simulink model "data_acquisition"  (R2023b)
settings: Solver=FixedStepDiscrete  StartTime=0.0  StopTime=Inf  RelTol=1e-3  EnableMultiTasking=on
libraries: c2802xlib x3
settings Model: SimulationMode=external  ExtModeTrigDuration=8  Creator=Yamukelani  LastModifiedBy=yamzi
settings SolverCC: AutoInsertRateTranBlk=on
settings DataIOCC: LoggingToFile=on  LoggingFileName=C:\Users\yamzi\source_code\msc_research\rul_prediction\src\datasets\msc_rul_data.mat
settings OptimizationCC: UseDivisionForNetSlopeComputation=on  GainParamInheritBuiltInType=on  UseFloatMulNetSlope=on  DefaultUnderspecifiedDataType=single  EnhancedBackFolding=on  PassReuseOutputArgsAs=Individual arguments  EfficientFloat2IntCast=on  MaxStackSize=768  OptimizeBlockOrder=speed  DifferentSizesBufferReuse=on  OptimizationCustomize=off  EfficientTunableParamExpr=on
settings DebuggingCC: ParameterTunabilityLossMsg=error
settings HardwareCC: ProdBitPerChar=16  ProdBitPerInt=16  ProdBitPerPointer=32  ProdBitPerSizeT=32  ProdBitPerPtrDiffT=32  ProdLargestAtomicInteger=Integer  ProdLargestAtomicFloat=None  ProdWordSize=16  ProdLongLongMode=on  ProdHWDeviceType=Texas Instruments->C2000  TargetBitPerPointer=64  TargetBitPerSizeT=64  TargetBitPerPtrDiffT=64  TargetLongLongMode=on  TargetIntDivRoundTo=Zero  TargetEndianess=LittleEndian  TargetWordSize=64  TargetHWDeviceType=MATLAB Host  ProdEqTarget=off
settings ModelReferenceCC: ModelReferenceNumInstancesAllowed=Single
settings SFSimCC: SimUserIncludeDirs=C:\ti\c2000\C2000Ware_5_01_00_00\device_support\f2802x\headers\include\  SimParseCustomCode=off  MATLABDynamicMemAlloc=off
settings SFSimCC: SimCustomHeaderCode=|
  | #ifdef MATLAB_MEX_FILE /*
  | /*Simulation behaviour */
  | #else
  | /*Code genration behavior*/
  | #include "DSP28x_Project.h"
  | #include "F2802x_Device.h"
  | #endif
settings RTWCC: Description=Embedded Coder  SystemTargetFile=ert.tlc  HardwareBoard=TI Piccolo F2802x  TemplateMakefile=ert_default_tmf  GenerateReport=on  CustomInclude=C:\ti\c2000\C2000Ware_5_01_00_00\device_support\f2802x\headers\include  CustomSource=C:\ti\c2000\C2000Ware_5_01_00_00\device_support\f2802x\common\source  CustomDefine=cregister=  Toolchain=Texas Instruments Code Composer Studio (C2000)  LaunchReport=on  CodeProfilingSaveOptions=MetricsOnly
settings RTWCC: CustomHeaderCode=|
  | #ifdef MATLAB_MEX_FILE /*
  | /*Simulation behaviour */
  | #else
  | /*Code genration behavior*/
  | #include "DSP28x_Project.h"
  | #include "F2802x_Device.h"
  | #endif
settings RTWCC: CustomInitializer=|
  | #ifndef MATLAB_MEX_FILE
  | #include "F2802x_Device.h"
  | #endif
settings CodeAppCC: ForceParamTrailComments=on  IgnoreCustomStorageClasses=off  OperatorAnnotations=on  SimulinkDataObjDesc=on  SFDataObjDesc=on  InsertBlockDesc=on
settings ERTTargetCC: ExtModeTransport=4  ExtModeStaticAlloc=on  ExtModeAutomaticAllocSize=off  ExtModeStaticAllocSize=500  ExtModeMexFile=ext_xcp  ExtModeIntrfLevel=Level2 - Open

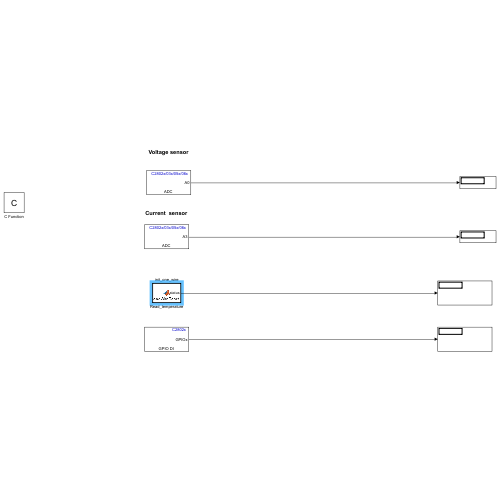
[thumbnail: Simulink's stored preview of the top-level diagram]
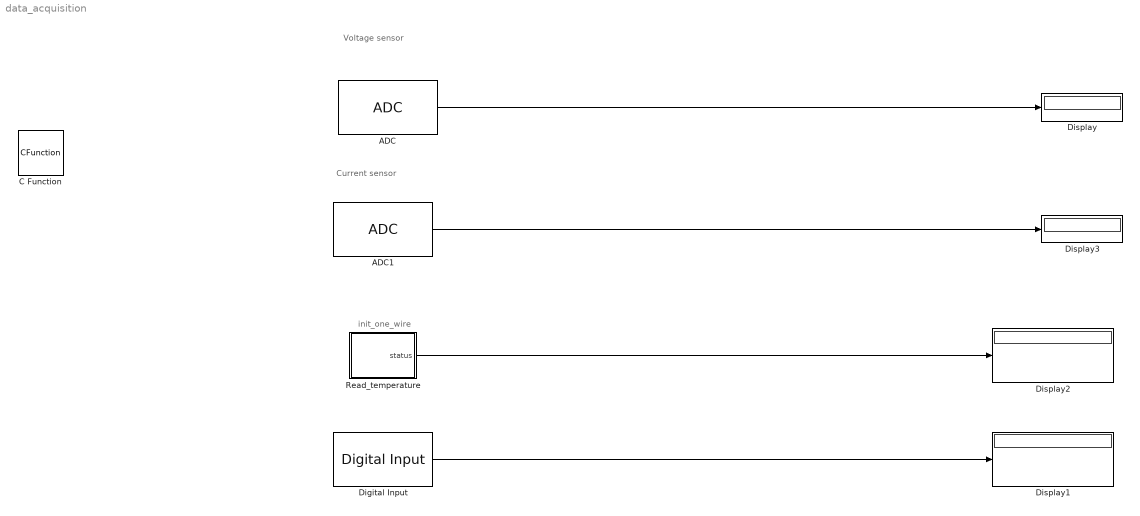
== system data_acquisition ==
  note: init_one_wire
  note: Current sensor
  note: Voltage sensor
  ADC : c2802xlib/ADC  blkParamProc=C2000  ADCModule=1  samplingMode=Single sample mode  ADCResolution=12-bit (Single-ended input)  useSOC1=SOC0  useSOC2=SOC0_SOC1  SOCAcquisitionWindow=7  SOCTriggerSource=CPU0_TINT0n  SOCInterruptTrigger=No ADCINT  Ts=0.005  dType=uint16  postInterrupt=off  interruptSel=ADCINT1  ADCINTContinuous=on  endma=off  chdma=1  conv1=ADCINA0  conv2=ADCINA0 and ADCINB0  conv1_Type4=ADCIN0  conv2_Type4=ADCIN0 and ADCIN1
  ADC1 : c2802xlib/ADC  blkParamProc=C2000  ADCModule=1  samplingMode=Single sample mode  ADCResolution=12-bit (Single-ended input)  useSOC1=SOC1  useSOC2=SOC0_SOC1  SOCAcquisitionWindow=7  SOCTriggerSource=CPU0_TINT0n  SOCInterruptTrigger=No ADCINT  Ts=0.005  dType=uint16  postInterrupt=off  interruptSel=ADCINT1  ADCINTContinuous=on  endma=off  chdma=1  conv1=ADCINA3  conv2=ADCINA0 and ADCINB0  conv1_Type4=ADCIN0  conv2_Type4=ADCIN0 and ADCIN1
  C Function : CFunction
  Digital Input : c2802xlib/Digital Input  GPIO_Number=GPIO0~GPIO7  GPIO_Bit0=on  GPIO_Bit1=off  GPIO_Bit2=off  GPIO_Bit3=off  GPIO_Bit4=off  GPIO_Bit5=off  GPIO_Bit6=off  GPIO_Bit7=off  sampleTime=0.1  dataType=auto  GPIO_Bit0_Qualification=Sync to SYSCLKOUT  GPIO_Bit1_Qualification=Sync to SYSCLKOUT  GPIO_Bit2_Qualification=Sync to SYSCLKOUT  GPIO_Bit3_Qualification=Sync to SYSCLKOUT  GPIO_Bit4_Qualification=Sync to SYSCLKOUT  GPIO_Bit5_Qualification=Sync to SYSCLKOUT  GPIO_Bit6_Qualification=Sync to SYSCLKOUT  GPIO_Bit7_Qualification=Sync to SYSCLKOUT  Qualification_Period=-1
  Display{,1..3} (4 alike) : Display
  Read_temperature : MATLAB Function  TreatAsAtomicUnit=on
  wires:
  ADC/1 -> Display/1
  ADC1/1 -> Display3/1
  Read_temperature/1(status) -> Display2/1
  Digital Input/1 -> Display1/1

== matlab function data_acquisition/Read_temperature ==
  data: status output
function status = oneWireReset()
    % Preinitialize status with a known type and size
    status = int32(0);  % Assuming status is an integer
    
    % Include necessary header files
    %coder.cinclude('F2802x_Device.h');

    % Set GPIO pin as output and drive it low
    coder.ceval('EALLOW'); % Enable write access to protected registers
    coder.ceval('GpioCtrlRegs.GPAMUX1.bit.GPIO0 = 0;'); % Configure as GPIO
    coder.ceval('GpioCtrlRegs.GPADIR.bit.GPIO0 = 1;'); % Set as output
    coder.ceval('GpioDataRegs.GPACLEAR.bit.GPIO0 = 1;'); % Drive low
    pause(0.00048); % 480 us delay
    
    % Release the bus and wait for presence pulse
    coder.ceval('GpioCtrlRegs.GPADIR.bit.GPIO0 = 0;'); % Set as input
    pause(0.00007); % 70 us delay
    status = coder.ceval('GpioDataRegs.GPADAT.bit.GPIO0'); % Read presence
    pause(0.00041); % 410 us delay
end
